simulink model "FOSWEC_Surge"  (R2015b)
settings: Solver=ode4  StartTime=0  StopTime=10  FixedStep=0.05  RelTol=1e-3
undefined symbols (not defined in the file or in its folder): body, constraint, mooring
libraries: WECSim_Lib x16
settings Model: Creator=cmichel  LastModifiedBy=kmruehl
settings DataIOCC: SaveFormat=Array
settings DebuggingCC: SolverPrmCheckMsg=warning
settings HardwareCC: ProdBitPerPointer=32  ProdLargestAtomicFloat=None  ProdIntDivRoundTo=Undefined  ProdEndianess=Unspecified  ProdWordSize=32  ProdHWDeviceType=32-bit Generic
settings GRTTargetCC: GeneratePreprocessorConditionals=Disable all
settings ConfigComp: CovModelRefEnable=Off  CovSFcnEnable=off

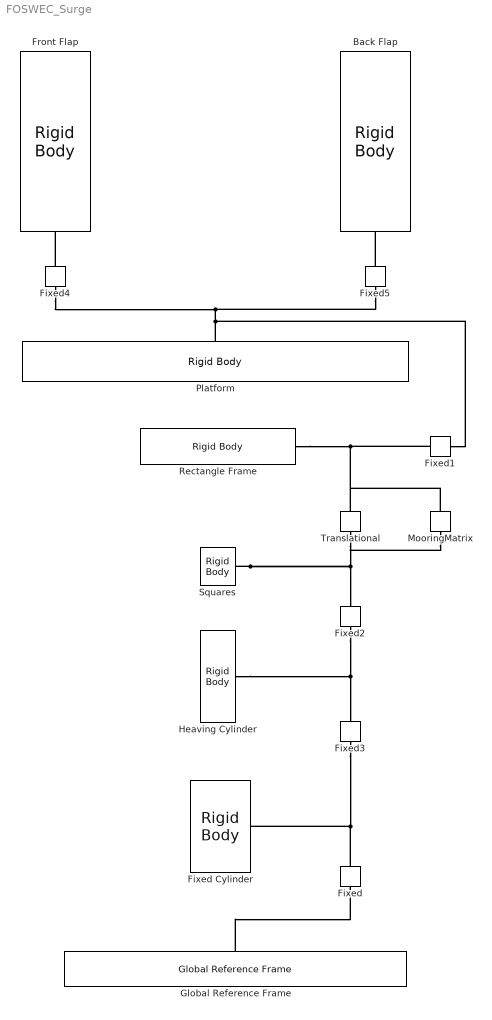
== system FOSWEC_Surge ==
  Back Flap : WECSim_Lib/Body Elements/Rigid Body  body=body(1)
      settings: AttributesFormatString=%<body>
  Fixed : WECSim_Lib/Constraints/Fixed  constraint=constraint(5)
      settings: AttributesFormatString=%<constraint>
  Fixed Cylinder : WECSim_Lib/Body Elements/Rigid Body  body=body(7)
      settings: AttributesFormatString=%<body>
  Fixed1 : WECSim_Lib/Constraints/Fixed  constraint=constraint(1)
      settings: AttributesFormatString=%<constraint>
  Fixed2 : WECSim_Lib/Constraints/Fixed  constraint=constraint(3)
      settings: AttributesFormatString=%<constraint>
  Fixed3 : WECSim_Lib/Constraints/Fixed  constraint=constraint(4)
      settings: AttributesFormatString=%<constraint>
  Fixed4 : WECSim_Lib/Constraints/Fixed  constraint=constraint(6)
      settings: AttributesFormatString=%<constraint>
  Fixed5 : WECSim_Lib/Constraints/Fixed  constraint=constraint(7)
      settings: AttributesFormatString=%<constraint>
  Front Flap : WECSim_Lib/Body Elements/Rigid Body  body=body(2)
      settings: AttributesFormatString=%<body>
  Global Reference Frame : WECSim_Lib/Frames/Global Reference Frame  waves=waves  simu=simu
  Heaving Cylinder : WECSim_Lib/Body Elements/Rigid Body  body=body(6)
      settings: AttributesFormatString=%<body>
  MooringMatrix : WECSim_Lib/Moorings/MooringMatrix  mooring=mooring(1)
      settings: AttributesFormatString=%<mooring>
  Platform : WECSim_Lib/Body Elements/Rigid Body  body=body(3)
      settings: AttributesFormatString=%<body>
  Rectangle Frame : WECSim_Lib/Body Elements/Rigid Body  body=body(4)
      settings: AttributesFormatString=%<body>
  Squares : WECSim_Lib/Body Elements/Rigid Body  body=body(5)
      settings: AttributesFormatString=%<body>
  Translational : WECSim_Lib/Constraints/Translational  constraint=constraint(2)
      settings: AttributesFormatString=%<constraint>
  connections:
  Fixed4/RConn1 -- Front Flap/RConn1
  Fixed5/RConn1 -- Back Flap/RConn1
  Platform/RConn1 -- Fixed1/RConn1 -- Fixed5/LConn1 -- Fixed4/LConn1
  Global Reference Frame/RConn1 -- Fixed/LConn1
  Squares/RConn1 -- MooringMatrix/RConn1 -- Translational/LConn1 -- Fixed2/RConn1
  Rectangle Frame/RConn1 -- MooringMatrix/LConn1 -- Translational/RConn1 -- Fixed1/LConn1
  Fixed2/LConn1 -- Heaving Cylinder/RConn1 -- Fixed3/RConn1
  Fixed3/LConn1 -- Fixed Cylinder/RConn1 -- Fixed/RConn1
